simulink library "INT_RmtAPP_SelSig"  (R2016b)
settings: Solver=VariableStepAuto  StartTime=0.0  StopTime=10.0  RelTol=1e-3
settings Model: Creator=bianxuyin  LastModifiedBy=bianxuyin

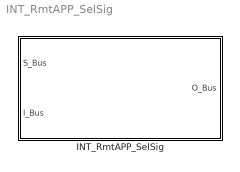
== system INT_RmtAPP_SelSig ==
  INT_RmtAPP_SelSig : Subsystem

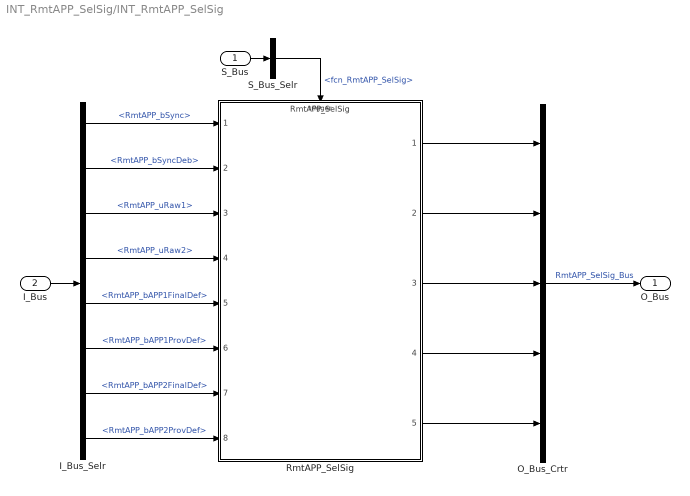
== system INT_RmtAPP_SelSig/INT_RmtAPP_SelSig ==
  S_Bus : Inport
  I_Bus : Inport  Port=2
  I_Bus_Selr : BusSelector  OutputSignals=RmtAPP_bSync,RmtAPP_bSyncDeb,RmtAPP_uRaw1,RmtAPP_uRaw2,RmtAPP_bAPP1FinalDef,RmtAPP_bAPP1ProvDef,RmtAPP_bAPP2FinalDef,RmtAPP_bAPP2ProvDef
  O_Bus_Crtr : BusCreator  Inputs=5
  RmtAPP_SelSig : ModelReference  ModelNameDialog=RmtAPP_SelSig  SimulationMode=Normal  ModelReferenceVersion=1.6  TriggerPortName=function  TriggerPortTriggerType=function-call  TriggerPortStatesWhenEnabling=held
  S_Bus_Selr : BusSelector  OutputSignals=fcn_RmtAPP_SelSig
  O_Bus : Outport
  wires:
  S_Bus_Selr/1 -> RmtAPP_SelSig/Trigger  "<fcn_RmtAPP_SelSig>"
  S_Bus/1 -> S_Bus_Selr/1
  I_Bus/1 -> I_Bus_Selr/1
  I_Bus_Selr/1 -> RmtAPP_SelSig/1  "<RmtAPP_bSync>"
  I_Bus_Selr/2 -> RmtAPP_SelSig/2  "<RmtAPP_bSyncDeb>"
  I_Bus_Selr/3 -> RmtAPP_SelSig/3  "<RmtAPP_uRaw1>"
  I_Bus_Selr/4 -> RmtAPP_SelSig/4  "<RmtAPP_uRaw2>"
  I_Bus_Selr/5 -> RmtAPP_SelSig/5  "<RmtAPP_bAPP1FinalDef>"
  I_Bus_Selr/6 -> RmtAPP_SelSig/6  "<RmtAPP_bAPP1ProvDef>"
  I_Bus_Selr/7 -> RmtAPP_SelSig/7  "<RmtAPP_bAPP2FinalDef>"
  I_Bus_Selr/8 -> RmtAPP_SelSig/8  "<RmtAPP_bAPP2ProvDef>"
  O_Bus_Crtr/1 -> O_Bus/1  "RmtAPP_SelSig_Bus"
  RmtAPP_SelSig/1 -> O_Bus_Crtr/1
  RmtAPP_SelSig/2 -> O_Bus_Crtr/2
  RmtAPP_SelSig/3 -> O_Bus_Crtr/3
  RmtAPP_SelSig/4 -> O_Bus_Crtr/4
  RmtAPP_SelSig/5 -> O_Bus_Crtr/5
